simulink library "tradSpoolingController_ul"  (R2018b)
settings: Solver=VariableStepAuto  StartTime=0.0  StopTime=10.0  RelTol=1e-3
undefined symbols (not defined in the file or in its folder): pathCtrl
libraries: firstOrderFilter_ul x1
settings Model: Creator=James Reed  LastModifiedBy=mcobb

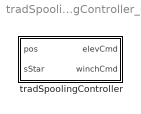
== system tradSpoolingController_ul ==
  tradSpoolingController : Subsystem

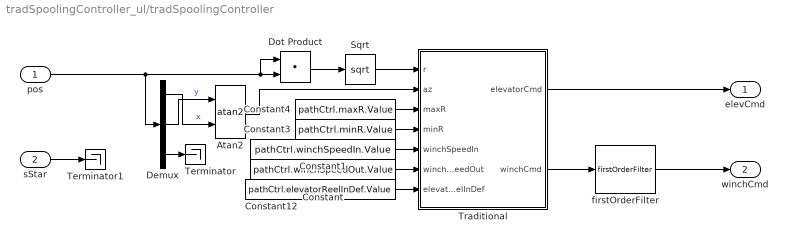
== system tradSpoolingController_ul/tradSpoolingController ==
  "pos " : Inport
  "sStar " : Inport  Port=2
  Atan2 : Trigonometry  Operator=atan2
  Constant : Constant  Value=pathCtrl.winchSpeedOut.Value
  Constant1 : Constant  Value=pathCtrl.winchSpeedIn.Value
  Constant12 : Constant  Value=pathCtrl.elevatorReelInDef.Value
  Constant3 : Constant  Value=pathCtrl.minR.Value
  Constant4 : Constant  Value=pathCtrl.maxR.Value
  Demux : Demux  Outputs=3
  Dot Product : DotProduct  InputSameDT=on  OutDataTypeStr=Inherit: Inherit via internal rule
  Sqrt : Sqrt  SaturateOnIntegerOverflow=on
  Terminator : Terminator
  Terminator1 : Terminator
  Traditional : Stateflow chart  TreatAsAtomicUnit=on
  firstOrderFilter : firstOrderFilter_ul/firstOrderFilter  tau=1  ic=0
  elevCmd : Outport
  "winchCmd " : Outport  Port=2
  wires:
  Traditional/1(elevatorCmd) -> elevCmd/1
  Traditional/2(winchCmd) -> firstOrderFilter/1
  firstOrderFilter/1 -> "winchCmd "/1
  "pos "/1 -> Demux/1, Dot Product/2, Dot Product/1
  "sStar "/1 -> Terminator1/1
  Constant4/1 -> Traditional/3(maxR)
  Constant3/1 -> Traditional/4(minR)
  Constant/1 -> Traditional/6(winchSpeedOut)
  Constant1/1 -> Traditional/5(winchSpeedIn)
  Constant12/1 -> Traditional/7(elevatorReelInDef)
  Demux/3 -> Terminator/1
  Sqrt/1 -> Traditional/1(r)
  Atan2/1 -> Traditional/2(az)
  Demux/1 -> Atan2/2  "x"
  Demux/2 -> Atan2/1  "y"
  Dot Product/1 -> Sqrt/1

== stateflow chart tradSpoolingController_ul/tradSpoolingController/Traditional ==
  state SpoolOut
    entry:
    winchCmd = winchSpeedOut;
    elevatorCmd = 0;
  state SpoolIn
    winchCmd = winchSpeedIn;
    elevatorCmd = elevatorReelInDef;
  (default) -> SpoolIn
  SpoolOut -> SpoolIn : [r > maxR ]
  SpoolIn -> SpoolOut : [r < minR]
  data: elevatorCmd output; r input; az input; winchCmd output; maxR input; minR input; winchSpeedIn input; winchSpeedOut input; elevatorReelInDef input
